simulink subsystem "SupervisoryControlSubsystem"  (R2023b)
settings: Solver=VariableStepAuto  StartTime=0.0  StopTime=10.0  RelTol=1e-3
settings Model: Creator=FRESH  LastModifiedBy=FRESH

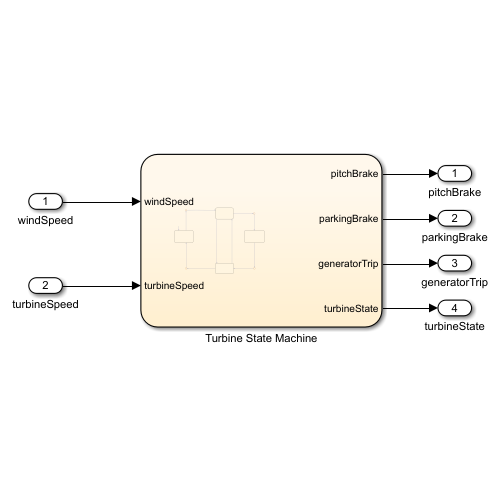
[thumbnail: Simulink's stored preview of the top-level diagram]
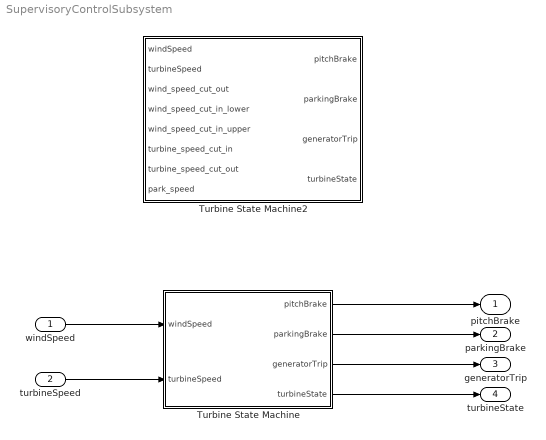
== system SupervisoryControlSubsystem ==
  windSpeed : Inport
  turbineSpeed : Inport  Port=2  OutDataTypeStr=double
  Turbine State Machine : Stateflow chart  TreatAsAtomicUnit=on
  Turbine State Machine2 : Stateflow chart  TreatAsAtomicUnit=on
      settings: PortSchema="{\"entries\":[{\"content\":{\"sides\":[{\"content\":{\"connectorIds\":[\"In1\",\"In2\",\"In4\",\"In3\",\"In5\",\"In6\",\"In7\",\"In8\"]},\"type\":\"ConnectorPlacement.EquallySpacedRectSide\",\"uuid\":\"10a1cf55-0e20-460b-8e2f-c1d1c7100ee9\"},{\"content\":{\"connectorIds\":[\"Out1\",\"Out2\",\"Out3\",\"Out4\"],\"side\":\"RIGHT\"},\"type\":\"ConnectorPlacement.EquallySpacedRectSide\",\"uuid\":\"a43f0466-98a7-49ac-bcbd-d1bb9fb5f160\"},{\"content\":{\"side\":\"TOP\"},\"type\":\"ConnectorPlacement.EquallySpacedRectSide\",\"uuid\":\"3d1c4b49-f5d5-4f3a-84f4-16750dfb675c\"}]},\"type\":\"ConnectorPlacement.EquallySpacedConnector\",\"uuid\":\"8e8882b2-d24e-4e45-9809-d94a40d36bf7\"}],\"packageUris\":[\"http://schema.mathworks.com/mf0/Connector/R2020b\"],\"version\":\"1.0\"}"
  pitchBrake : Outport
  parkingBrake : Outport  Port=2
  generatorTrip : Outport  Port=3
  turbineState : Outport  Port=4
  wires:
  windSpeed/1 -> Turbine State Machine/1(windSpeed)
  turbineSpeed/1 -> Turbine State Machine/2(turbineSpeed)
  Turbine State Machine/1(pitchBrake) -> pitchBrake/1
  Turbine State Machine/2(parkingBrake) -> parkingBrake/1
  Turbine State Machine/3(generatorTrip) -> generatorTrip/1
  Turbine State Machine/4(turbineState) -> turbineState/1

== stateflow chart SupervisoryControlSubsystem/Turbine State Machine2 ==
  state Startup
    entry: parkingBrake = 0;
    generatorTrip = 1;
    pitchBrake = 0;
    turbineState = 1;
  state ParkBrake
    entry: parkingBrake = 1;
    generatorTrip = 1;
    pitchBrake = 1;
    turbineState = 0;
  state Generating
    entry: parkingBrake = 0;
    generatorTrip = 0;
    pitchBrake = 0;
    turbineState = 2;
  state PitchBrake
    entry: parkingBrake = 0;
    generatorTrip = 0;
    pitchBrake = 1;
    turbineState = 3;
  (junction 42) -> Startup : [duration(windSpeed>wind_speed_cut_in_lower)>0.10&&duration(windSpeed<wind_speed_cut_out)>0.10]
  ParkBrake -> (junction 42)
  Startup -> (junction 52) [order 1] : [duration(turbineSpeed>turbine_speed_cut_in)>0.10]
  (junction 52) -> Generating
  Startup -> PitchBrake [order 2] : [duration(windSpeed<wind_speed_cut_in_lower)>1.0 || duration(windSpeed>wind_speed_cut_out)>1.0]
  PitchBrake -> Startup [order 2] : [duration(windSpeed<=wind_speed_cut_in_upper)>2.0 && duration(windSpeed>wind_speed_cut_in_lower)>2.0 && duration(turbineSpeed<turbine_speed_cut_in)>2.0]
  (default) -> ParkBrake
  (junction 45) -> ParkBrake
  Generating -> (junction 55) : [duration(windSpeed<wind_speed_cut_in_lower)>0.10||duration(windSpeed>wind_speed_cut_out)>0.10||duration(turbineSpeed>turbine_speed_cut_out)>0.10||duration(turbineSpeed<turbine_speed_cut_in)>0.10]
  (junction 55) -> PitchBrake
  PitchBrake -> (junction 45) [order 1] : [duration(turbineSpeed<=park_speed)>0.10]
  data: windSpeed input; turbineSpeed input; pitchBrake output; parkingBrake output; generatorTrip output; turbineState output; wind_speed_cut_in_lower input; wind_speed_cut_out input; wind_speed_cut_in_upper input; turbine_speed_cut_in input; turbine_speed_cut_out input; park_speed input

== stateflow chart SupervisoryControlSubsystem/Turbine State Machine ==
  state Startup
    entry: parkingBrake = 0;
    generatorTrip = 1;
    pitchBrake = 0;
    turbineState = 1;
  state Generating
    entry: parkingBrake = 0;
    generatorTrip = 0;
    pitchBrake = 0;
    turbineState = 2;
  state ParkBrake
    entry: parkingBrake = 1;
    generatorTrip = 1;
    pitchBrake = 1;
    turbineState = 0;
  state PitchBrake
    entry: parkingBrake = 0;
    generatorTrip = 0;
    pitchBrake = 1;
    turbineState = 3;
  (junction 37) -> Startup : [duration(windSpeed>...
      | wind_speed_cut_in_lower)>0.10...
      | &&duration(windSpeed<...
      | wind_speed_cut_out)>0.10]
  ParkBrake -> (junction 37)
  Startup -> (junction 41) [order 1] : [duration(turbineSpeed>...
      | turbine_speed_cut_in)>0.10]
  (junction 41) -> Generating
  Startup -> PitchBrake [order 2] : [duration(windSpeed<...
      | wind_speed_cut_in_lower)>1.0...
      | ||duration(windSpeed>...
      | wind_speed_cut_out)>1.0]
  PitchBrake -> Startup [order 2] : [duration(windSpeed<=...
      | wind_speed_cut_in_upper)>2.0...
      | && duration(windSpeed>...
      | wind_speed_cut_in_lower)>2.0...
      | && duration(turbineSpeed<...
      | turbine_speed_cut_in)>2.0]
  (default) -> ParkBrake
  Generating -> (junction 43) : [duration(windSpeed<...
      | wind_speed_cut_in_lower)>0.10...
      | ||duration(windSpeed>...
      | wind_speed_cut_out)>0.10...
      | ||duration(turbineSpeed>...
      | turbine_speed_cut_out)>0.10...
      | ||duration(turbineSpeed<...
      | turbine_speed_cut_in)>0.10]
  (junction 39) -> ParkBrake
  PitchBrake -> (junction 39) [order 1] : [duration(turbineSpeed<=...
      | park_speed)>0.10]
  (junction 43) -> PitchBrake
  data: pitchBrake output double; windSpeed input; turbineSpeed input; parkingBrake output double; generatorTrip output double; wind_speed_cut_in_lower local double =vWindCutInLower; turbine_speed_cut_in local double =wTurbineCutIn; turbineState output double; wind_speed_cut_out local double =vWindCutOut; wind_speed_cut_in_upper local double =vWindCutInUpper; turbine_speed_cut_out local double =wTurbineCutOut; park_speed constant double =wTurbinePark
